simulink model "Energy_Release_System"  (R2022b)
settings: Solver=FixedStepAuto  StartTime=0.0  StopTime=2000  FixedStep=1  RelTol=1e-3
model workspace (MAT data in the model file):
  P0 = 13000
  T0 = 700
  m0 = 30000000
settings Model: Creator=Crapon  LastModifiedBy=Crapon

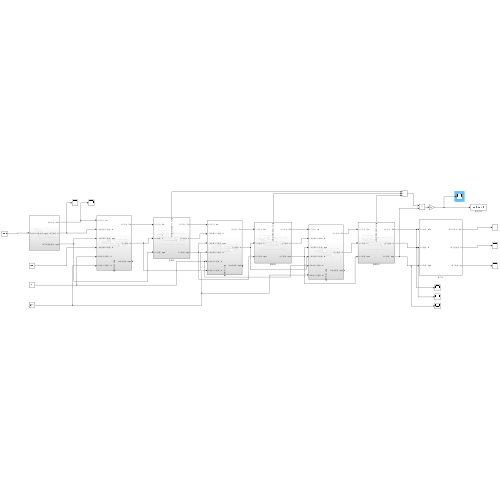
[thumbnail: Simulink's stored preview of the top-level diagram]
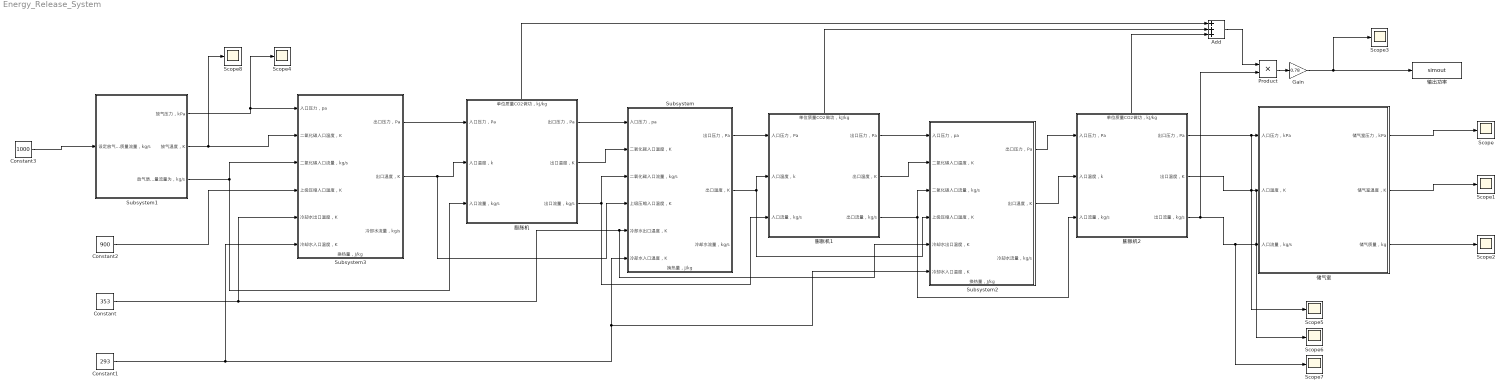
== system Energy_Release_System ==
  Add : Sum  Inputs=+++
  Constant : Constant  Value=353
  Constant1 : Constant  Value=293
  Constant2 : Constant  Value=900
  Constant3 : Constant  Value=1000
  Gain : Gain  Gain=0.78
  Product : Product
  Scope{,1..8} (9 alike) : Scope
  Subsystem : Subsystem
      settings: PortSchema="{\"entries\":[{\"content\":{\"sides\":[{\"content\":{\"connectorIds\":[\"In1\",\"In2\",\"In3\",\"In4\",\"In5\",\"In6\"]},\"type\":\"ConnectorPlacement.EquallySpacedRectSide\",\"uuid\":\"005acfd8-ea89-4894-a254-a05d71797730\"},{\"content\":{\"connectorIds\":[\"Out1\",\"Out2\",\"Out3\"],\"side\":\"RIGHT\"},\"type\":\"ConnectorPlacement.EquallySpacedRectSide\",\"uuid\":\"e66330f7-ec29-462a-8cb5-548756672f09\"},{\"content\":{\"connectorIds\":[],\"side\":\"TOP\"},\"type\":\"ConnectorPlacement.EquallySpacedRectSide\",\"uuid\":\"f5e02eef-e82e-41bc-9a16-8c3a3dd05456\"},{\"content\":{\"connectorIds\":[\"Out4\"],\"side\":\"BOTTOM\"},\"type\":\"ConnectorPlacement.EquallySpacedRectSide\",\"uuid\":\"90480476-9594-4c11-8a2f-3b3d9fc35a98\"}]},\"type\":\"ConnectorPlacement.EquallySpacedConnector\",\"uuid\":\"2499ac2c-0893-45bb-b507-b450c1c8eb76\"}],\"packageUris\":[\"http://schema.mathworks.com/mf0/Connector/R2020b\"],\"version\":\"1.0\"}"
  Subsystem1 : Subsystem
  Subsystem2 : Subsystem
      settings: PortSchema="{\"entries\":[{\"content\":{\"sides\":[{\"content\":{\"connectorIds\":[\"In1\",\"In2\",\"In3\",\"In4\",\"In5\",\"In6\"]},\"type\":\"ConnectorPlacement.EquallySpacedRectSide\",\"uuid\":\"005acfd8-ea89-4894-a254-a05d71797730\"},{\"content\":{\"connectorIds\":[\"Out1\",\"Out2\",\"Out3\"],\"side\":\"RIGHT\"},\"type\":\"ConnectorPlacement.EquallySpacedRectSide\",\"uuid\":\"e66330f7-ec29-462a-8cb5-548756672f09\"},{\"content\":{\"connectorIds\":[],\"side\":\"TOP\"},\"type\":\"ConnectorPlacement.EquallySpacedRectSide\",\"uuid\":\"f5e02eef-e82e-41bc-9a16-8c3a3dd05456\"},{\"content\":{\"connectorIds\":[\"Out4\"],\"side\":\"BOTTOM\"},\"type\":\"ConnectorPlacement.EquallySpacedRectSide\",\"uuid\":\"90480476-9594-4c11-8a2f-3b3d9fc35a98\"}]},\"type\":\"ConnectorPlacement.EquallySpacedConnector\",\"uuid\":\"2499ac2c-0893-45bb-b507-b450c1c8eb76\"}],\"packageUris\":[\"http://schema.mathworks.com/mf0/Connector/R2020b\"],\"version\":\"1.0\"}"
  Subsystem3 : Subsystem
      settings: PortSchema="{\"entries\":[{\"content\":{\"sides\":[{\"content\":{\"connectorIds\":[\"In1\",\"In2\",\"In3\",\"In4\",\"In5\",\"In6\"]},\"type\":\"ConnectorPlacement.EquallySpacedRectSide\",\"uuid\":\"005acfd8-ea89-4894-a254-a05d71797730\"},{\"content\":{\"connectorIds\":[\"Out1\",\"Out2\",\"Out3\"],\"side\":\"RIGHT\"},\"type\":\"ConnectorPlacement.EquallySpacedRectSide\",\"uuid\":\"e66330f7-ec29-462a-8cb5-548756672f09\"},{\"content\":{\"connectorIds\":[],\"side\":\"TOP\"},\"type\":\"ConnectorPlacement.EquallySpacedRectSide\",\"uuid\":\"f5e02eef-e82e-41bc-9a16-8c3a3dd05456\"},{\"content\":{\"connectorIds\":[\"Out4\"],\"side\":\"BOTTOM\"},\"type\":\"ConnectorPlacement.EquallySpacedRectSide\",\"uuid\":\"90480476-9594-4c11-8a2f-3b3d9fc35a98\"}]},\"type\":\"ConnectorPlacement.EquallySpacedConnector\",\"uuid\":\"2499ac2c-0893-45bb-b507-b450c1c8eb76\"}],\"packageUris\":[\"http://schema.mathworks.com/mf0/Connector/R2020b\"],\"version\":\"1.0\"}"
  储气室 : Subsystem
  膨胀机 : Subsystem
      settings: PortSchema="{\"entries\":[{\"content\":{\"sides\":[{\"content\":{\"connectorIds\":[\"In1\",\"In2\",\"In3\"]},\"type\":\"ConnectorPlacement.EquallySpacedRectSide\",\"uuid\":\"af46db4a-1baf-47a9-bc8e-dce7f9faf651\"},{\"content\":{\"connectorIds\":[\"Out1\",\"Out2\",\"Out3\"],\"side\":\"RIGHT\"},\"type\":\"ConnectorPlacement.EquallySpacedRectSide\",\"uuid\":\"0ecd7e62-bca6-4a18-8bf4-9fc15378ff92\"},{\"content\":{\"connectorIds\":[\"Out4\"],\"side\":\"TOP\"},\"type\":\"ConnectorPlacement.EquallySpacedRectSide\",\"uuid\":\"ae3c27ab-cc75-4c7c-b9ef-cea9554166bd\"}]},\"type\":\"ConnectorPlacement.EquallySpacedConnector\",\"uuid\":\"4d6f15aa-483c-4043-8dfd-1170adfd8f34\"}],\"packageUris\":[\"http://schema.mathworks.com/mf0/Connector/R2020b\"],\"version\":\"1.0\"}"
  膨胀机1 : Subsystem
      settings: PortSchema="{\"entries\":[{\"content\":{\"sides\":[{\"content\":{\"connectorIds\":[\"In1\",\"In2\",\"In3\"]},\"type\":\"ConnectorPlacement.EquallySpacedRectSide\",\"uuid\":\"af46db4a-1baf-47a9-bc8e-dce7f9faf651\"},{\"content\":{\"connectorIds\":[\"Out1\",\"Out2\",\"Out3\"],\"side\":\"RIGHT\"},\"type\":\"ConnectorPlacement.EquallySpacedRectSide\",\"uuid\":\"0ecd7e62-bca6-4a18-8bf4-9fc15378ff92\"},{\"content\":{\"connectorIds\":[\"Out4\"],\"side\":\"TOP\"},\"type\":\"ConnectorPlacement.EquallySpacedRectSide\",\"uuid\":\"ae3c27ab-cc75-4c7c-b9ef-cea9554166bd\"}]},\"type\":\"ConnectorPlacement.EquallySpacedConnector\",\"uuid\":\"4d6f15aa-483c-4043-8dfd-1170adfd8f34\"}],\"packageUris\":[\"http://schema.mathworks.com/mf0/Connector/R2020b\"],\"version\":\"1.0\"}"
  膨胀机2 : Subsystem
      settings: PortSchema="{\"entries\":[{\"content\":{\"sides\":[{\"content\":{\"connectorIds\":[\"In1\",\"In2\",\"In3\"]},\"type\":\"ConnectorPlacement.EquallySpacedRectSide\",\"uuid\":\"af46db4a-1baf-47a9-bc8e-dce7f9faf651\"},{\"content\":{\"connectorIds\":[\"Out1\",\"Out2\",\"Out3\"],\"side\":\"RIGHT\"},\"type\":\"ConnectorPlacement.EquallySpacedRectSide\",\"uuid\":\"0ecd7e62-bca6-4a18-8bf4-9fc15378ff92\"},{\"content\":{\"connectorIds\":[\"Out4\"],\"side\":\"TOP\"},\"type\":\"ConnectorPlacement.EquallySpacedRectSide\",\"uuid\":\"ae3c27ab-cc75-4c7c-b9ef-cea9554166bd\"}]},\"type\":\"ConnectorPlacement.EquallySpacedConnector\",\"uuid\":\"4d6f15aa-483c-4043-8dfd-1170adfd8f34\"}],\"packageUris\":[\"http://schema.mathworks.com/mf0/Connector/R2020b\"],\"version\":\"1.0\"}"
  输出功率 : ToWorkspace  VariableName=simout  SaveFormat=Timeseries  SampleTime=-1
  wires:
  Subsystem3/1(出口压力，Pa) -> 膨胀机/1(入口压力，Pa)
  Subsystem3/2(出口温度，K) -> Subsystem/4(上级压缩入口温度，K), 膨胀机/2(入口温度，k)
  Subsystem1/3(放气质量流量为，kg/s) -> Subsystem3/3(二氧化碳入口流量，kg/s), 膨胀机/3(入口流量，kg/s)
  膨胀机/1(出口压力，Pa) -> Subsystem/1(入口压力，pa)
  膨胀机/2(出口温度，K) -> Subsystem/2(二氧化碳入口温度，K)
  膨胀机/3("  出口流量，kg/s") -> Subsystem/3(二氧化碳入口流量，kg/s), 膨胀机1/3(入口流量，kg/s)
  Subsystem/1(出口压力，Pa) -> 膨胀机1/1(入口压力，Pa)
  Subsystem/2(出口温度，K) -> Subsystem2/4(上级压缩入口温度，K), 膨胀机1/2(入口温度，k)
  膨胀机1/1(出口压力，Pa) -> Subsystem2/1(入口压力，pa)
  膨胀机1/2(出口温度，K) -> Subsystem2/2(二氧化碳入口温度，K)
  膨胀机1/3("  出口流量，kg/s") -> 膨胀机2/3(入口流量，kg/s), Subsystem2/3(二氧化碳入口流量，kg/s)
  Subsystem2/1(出口压力，Pa) -> 膨胀机2/1(入口压力，Pa)
  Subsystem2/2(出口温度，K) -> 膨胀机2/2(入口温度，k)
  膨胀机/4(单位质量CO2做功，kJ/kg) -> Add/1
  膨胀机1/4(单位质量CO2做功，kJ/kg) -> Add/2
  膨胀机2/1(出口压力，Pa) -> Scope5/1, 储气室/1(入口压力，kPa)
  膨胀机2/2(出口温度，K) -> Scope6/1, 储气室/2(入口温度，K)
  膨胀机2/3("  出口流量，kg/s") -> Product/2, Scope7/1, 储气室/3(入口流量，kg/s)
  储气室/3(储气质量，kg) -> Scope2/1
  储气室/2(储气室温度，K) -> Scope1/1
  储气室/1(储气室压力，kPa) -> Scope/1
  膨胀机2/4(单位质量CO2做功，kJ/kg) -> Add/3
  Add/1 -> Product/1
  Product/1 -> Gain/1
  Gain/1 -> Scope3/1, 输出功率/1
  Constant/1 -> Subsystem3/5(冷却水出口温度，K), Subsystem2/5(冷却水出口温度，K), Subsystem/5(冷却水出口温度，K)
  Constant1/1 -> Subsystem3/6(冷却水入口温度，K), Subsystem2/6(冷却水入口温度，K), Subsystem/6(冷却水入口温度，K)
  Constant2/1 -> Subsystem3/4(上级压缩入口温度，K)
  Subsystem1/1(放气压力，kPa) -> Scope4/1, Subsystem3/1(入口压力，pa)
  Subsystem1/2(放气温度，K) -> Scope8/1, Subsystem3/2(二氧化碳入口温度，K)
  Constant3/1 -> Subsystem1/1(设定放气质量流量，kg/s)

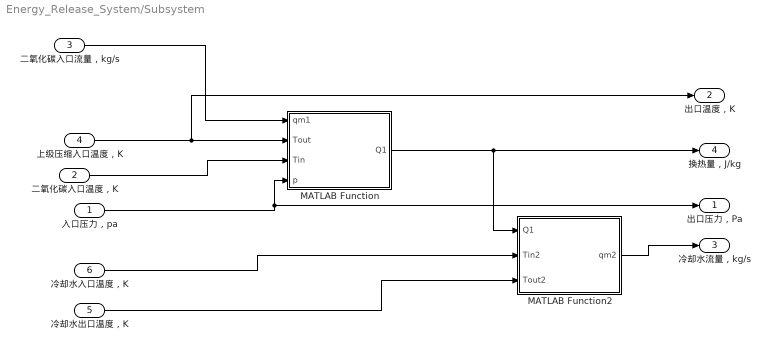
== system Energy_Release_System/Subsystem ==
  入口压力，pa : Inport
  二氧化碳入口温度，K : Inport  Port=2
  二氧化碳入口流量，kg/s : Inport  Port=3
  上级压缩入口温度，K : Inport  Port=4
  冷却水出口温度，K : Inport  Port=5
  冷却水入口温度，K : Inport  Port=6
  MATLAB Function : MATLAB Function  TreatAsAtomicUnit=on
  MATLAB Function2 : MATLAB Function  TreatAsAtomicUnit=on
  出口压力，Pa : Outport
  出口温度，K : Outport  Port=2
  冷却水流量，kg/s : Outport  Port=3
  换热量，J/kg : Outport  Port=4
  wires:
  MATLAB Function/1(Q1) -> 换热量，J/kg/1, MATLAB Function2/1(Q1)
  冷却水出口温度，K/1 -> MATLAB Function2/3(Tout2)
  冷却水入口温度，K/1 -> MATLAB Function2/2(Tin2)
  MATLAB Function2/1(qm2) -> 冷却水流量，kg/s/1
  二氧化碳入口温度，K/1 -> MATLAB Function/3(Tin)
  上级压缩入口温度，K/1 -> 出口温度，K/1, MATLAB Function/2(Tout)
  二氧化碳入口流量，kg/s/1 -> MATLAB Function/1(qm1)
  入口压力，pa/1 -> MATLAB Function/4(p), 出口压力，Pa/1

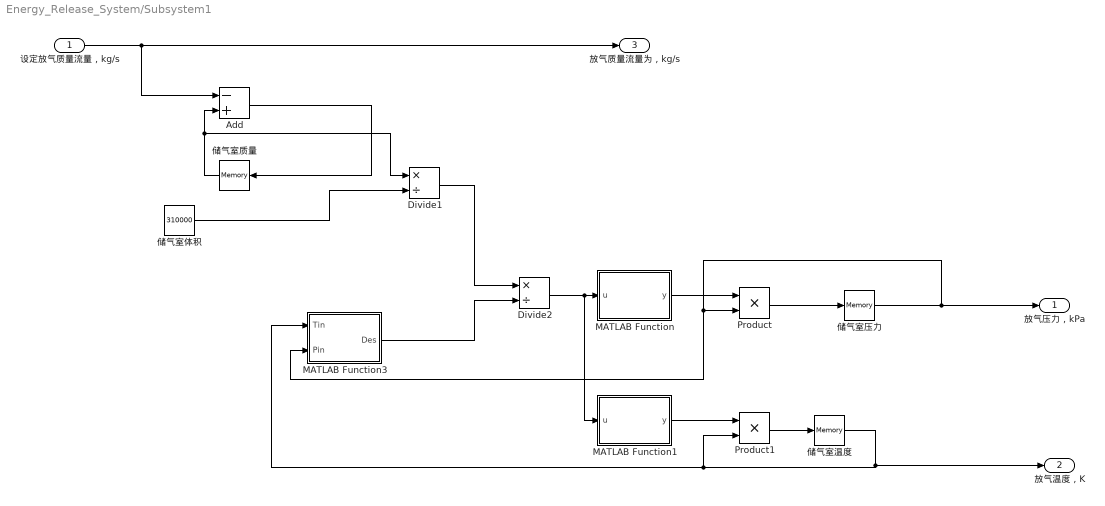
== system Energy_Release_System/Subsystem1 ==
  设定放气质量流量，kg/s : Inport
  Add : Sum  Inputs=-+
  Divide1 : Product  Inputs=*/
  Divide2 : Product  Inputs=*/
  MATLAB Function : MATLAB Function  TreatAsAtomicUnit=on
  MATLAB Function1 : MATLAB Function  TreatAsAtomicUnit=on
  MATLAB Function3 : MATLAB Function  TreatAsAtomicUnit=on
  Product : Product
  Product1 : Product
  储气室体积 : Constant  Value=310000
  储气室压力 : Memory  InitialCondition=P0
  储气室温度 : Memory  InitialCondition=T0
  储气室质量 : Memory  InitialCondition=m0
  放气压力，kPa : Outport
  放气温度，K : Outport  Port=2
  放气质量流量为，kg/s : Outport  Port=3
  wires:
  设定放气质量流量，kg/s/1 -> 放气质量流量为，kg/s/1, Add/1
  MATLAB Function3/1(Des) -> Divide2/2
  储气室质量/1 -> Divide1/1, Add/2
  Add/1 -> 储气室质量/1
  储气室体积/1 -> Divide1/2
  Divide1/1 -> Divide2/1
  Divide2/1 -> MATLAB Function1/1(u), MATLAB Function/1(u)
  储气室压力/1 -> Product/2, MATLAB Function3/2(Pin), 放气压力，kPa/1
  Product/1 -> 储气室压力/1
  MATLAB Function1/1(y) -> Product1/1
  Product1/1 -> 储气室温度/1
  储气室温度/1 -> MATLAB Function3/1(Tin), Product1/2, 放气温度，K/1
  MATLAB Function/1(y) -> Product/1

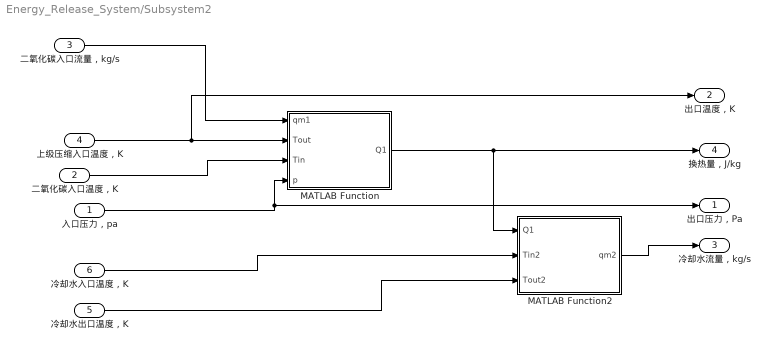
== system Energy_Release_System/Subsystem2 ==
  入口压力，pa : Inport
  二氧化碳入口温度，K : Inport  Port=2
  二氧化碳入口流量，kg/s : Inport  Port=3
  上级压缩入口温度，K : Inport  Port=4
  冷却水出口温度，K : Inport  Port=5
  冷却水入口温度，K : Inport  Port=6
  MATLAB Function : MATLAB Function  TreatAsAtomicUnit=on
  MATLAB Function2 : MATLAB Function  TreatAsAtomicUnit=on
  出口压力，Pa : Outport
  出口温度，K : Outport  Port=2
  冷却水流量，kg/s : Outport  Port=3
  换热量，J/kg : Outport  Port=4
  wires:
  入口压力，pa/1 -> 出口压力，Pa/1, MATLAB Function/4(p)
  二氧化碳入口流量，kg/s/1 -> MATLAB Function/1(qm1)
  上级压缩入口温度，K/1 -> MATLAB Function/2(Tout), 出口温度，K/1
  二氧化碳入口温度，K/1 -> MATLAB Function/3(Tin)
  MATLAB Function2/1(qm2) -> 冷却水流量，kg/s/1
  冷却水入口温度，K/1 -> MATLAB Function2/2(Tin2)
  冷却水出口温度，K/1 -> MATLAB Function2/3(Tout2)
  MATLAB Function/1(Q1) -> MATLAB Function2/1(Q1), 换热量，J/kg/1

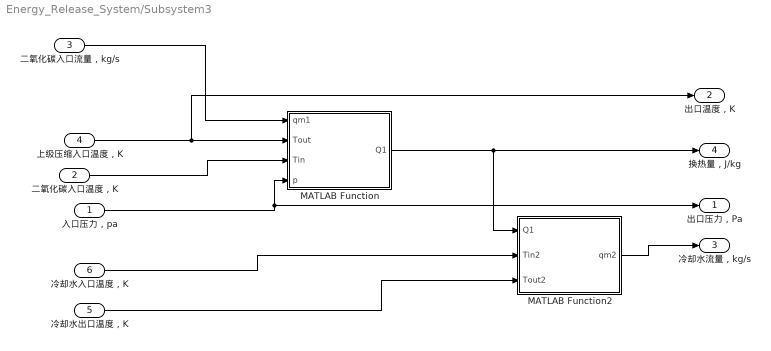
== system Energy_Release_System/Subsystem3 ==
  入口压力，pa : Inport
  二氧化碳入口温度，K : Inport  Port=2
  二氧化碳入口流量，kg/s : Inport  Port=3
  上级压缩入口温度，K : Inport  Port=4
  冷却水出口温度，K : Inport  Port=5
  冷却水入口温度，K : Inport  Port=6
  MATLAB Function : MATLAB Function  TreatAsAtomicUnit=on
  MATLAB Function2 : MATLAB Function  TreatAsAtomicUnit=on
  出口压力，Pa : Outport
  出口温度，K : Outport  Port=2
  冷却水流量，kg/s : Outport  Port=3
  换热量，J/kg : Outport  Port=4
  wires:
  入口压力，pa/1 -> 出口压力，Pa/1, MATLAB Function/4(p)
  二氧化碳入口流量，kg/s/1 -> MATLAB Function/1(qm1)
  上级压缩入口温度，K/1 -> MATLAB Function/2(Tout), 出口温度，K/1
  二氧化碳入口温度，K/1 -> MATLAB Function/3(Tin)
  MATLAB Function2/1(qm2) -> 冷却水流量，kg/s/1
  冷却水入口温度，K/1 -> MATLAB Function2/2(Tin2)
  冷却水出口温度，K/1 -> MATLAB Function2/3(Tout2)
  MATLAB Function/1(Q1) -> MATLAB Function2/1(Q1), 换热量，J/kg/1

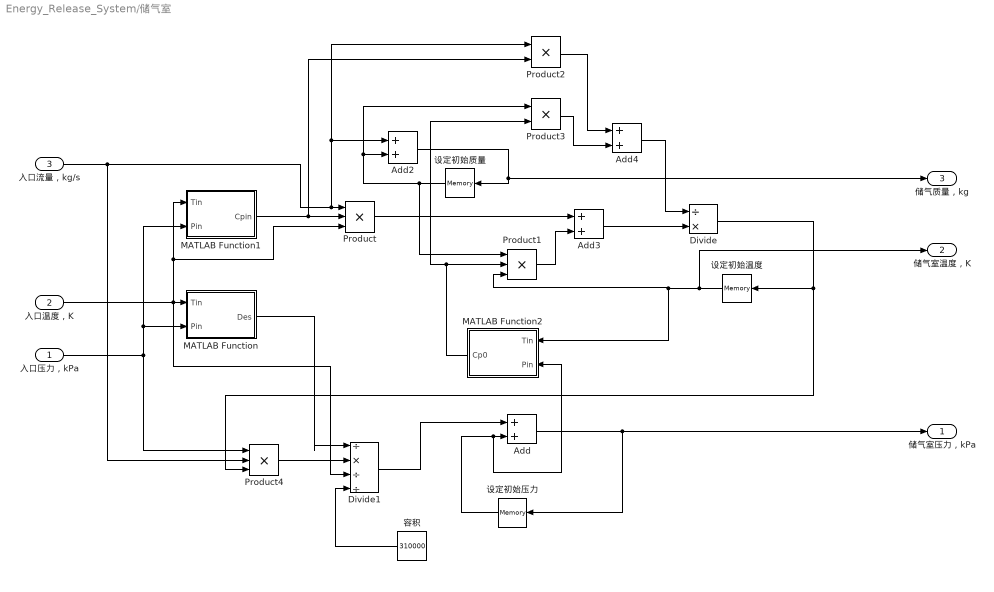
== system Energy_Release_System/储气室 ==
  入口压力，kPa : Inport
  入口温度，K : Inport  Port=2
  入口流量，kg/s : Inport  Port=3
  Add{,2..4} (4 alike) : Sum
  Divide : Product  Inputs=/*
  Divide1 : Product  Inputs=/*//
  MATLAB Function : MATLAB Function  TreatAsAtomicUnit=on
  MATLAB Function1 : MATLAB Function  TreatAsAtomicUnit=on
  MATLAB Function2 : MATLAB Function  TreatAsAtomicUnit=on
  Product : Product  Inputs=3
  Product1 : Product  Inputs=3
  Product2 : Product
  Product3 : Product
  Product4 : Product  Inputs=3
  容积 : Constant  Value=310000
  设定初始压力 : Memory  InitialCondition=100
  设定初始温度 : Memory  InitialCondition=300
  设定初始质量 : Memory  InitialCondition=320000
  储气室压力，kPa : Outport
  储气室温度，K : Outport  Port=2
  储气质量，kg : Outport  Port=3
  wires:
  入口流量，kg/s/1 -> Product4/2, Product2/1, Add2/1, Product/1
  设定初始质量/1 -> Product1/1, Product3/1, Add2/2
  Product2/1 -> Add4/1
  MATLAB Function1/1(Cpin) -> Product/2, Product2/2
  Product4/1 -> Divide1/2
  MATLAB Function2/1(Cp0) -> Product1/2, Product3/2
  Divide1/1 -> Add/1
  入口温度，K/1 -> MATLAB Function1/1(Tin), Product/3, MATLAB Function/1(Tin), Divide1/3
  Product1/1 -> Add3/2
  Add/1 -> 储气室压力，kPa/1, 设定初始压力/1
  入口压力，kPa/1 -> Product4/1, MATLAB Function1/2(Pin), MATLAB Function/2(Pin)
  Add4/1 -> Divide/1
  设定初始压力/1 -> MATLAB Function2/2(Pin), Add/2
  容积/1 -> Divide1/4
  Product3/1 -> Add4/2
  MATLAB Function/1(Des) -> Divide1/1
  Add3/1 -> Divide/2
  Product/1 -> Add3/1
  Divide/1 -> Product4/3, 设定初始温度/1
  Add2/1 -> 设定初始质量/1, 储气质量，kg/1
  设定初始温度/1 -> 储气室温度，K/1, MATLAB Function2/1(Tin), Product1/3

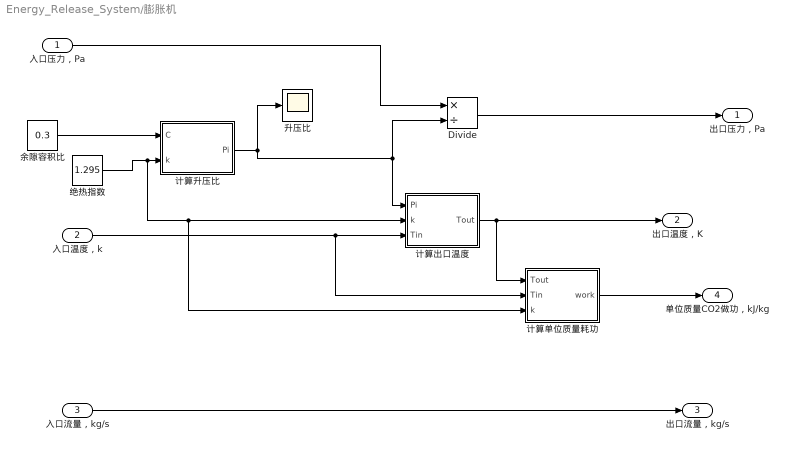
== system Energy_Release_System/膨胀机 ==
  入口压力，Pa : Inport
  入口温度，k : Inport  Port=2
  入口流量，kg/s : Inport  Port=3
  Divide : Product  Inputs=*/
  余隙容积比 : Constant  Value=0.3
  升压比 : Scope
  绝热指数 : Constant  Value=1.295
  计算出口温度 : MATLAB Function  TreatAsAtomicUnit=on
  计算升压比 : MATLAB Function  TreatAsAtomicUnit=on
  计算单位质量耗功 : MATLAB Function  TreatAsAtomicUnit=on
  出口压力，Pa : Outport
  出口温度，K : Outport  Port=2
  "  出口流量，kg/s" : Outport  Port=3
  单位质量CO2做功，kJ/kg : Outport  Port=4
  wires:
  余隙容积比/1 -> 计算升压比/1(C)
  入口压力，Pa/1 -> Divide/1
  绝热指数/1 -> 计算单位质量耗功/3(k), 计算出口温度/2(k), 计算升压比/2(k)
  Divide/1 -> 出口压力，Pa/1
  计算单位质量耗功/1(work) -> 单位质量CO2做功，kJ/kg/1
  计算升压比/1(Pi) -> Divide/2, 计算出口温度/1(Pi), 升压比/1
  入口温度，k/1 -> 计算单位质量耗功/2(Tin), 计算出口温度/3(Tin)
  计算出口温度/1(Tout) -> 出口温度，K/1, 计算单位质量耗功/1(Tout)
  入口流量，kg/s/1 -> "  出口流量，kg/s"/1

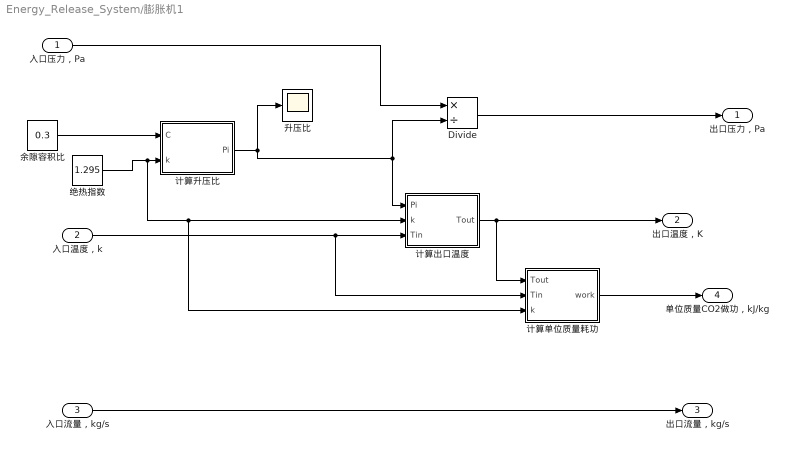
== system Energy_Release_System/膨胀机1 ==
  入口压力，Pa : Inport
  入口温度，k : Inport  Port=2
  入口流量，kg/s : Inport  Port=3
  Divide : Product  Inputs=*/
  余隙容积比 : Constant  Value=0.3
  升压比 : Scope
  绝热指数 : Constant  Value=1.295
  计算出口温度 : MATLAB Function  TreatAsAtomicUnit=on
  计算升压比 : MATLAB Function  TreatAsAtomicUnit=on
  计算单位质量耗功 : MATLAB Function  TreatAsAtomicUnit=on
  出口压力，Pa : Outport
  出口温度，K : Outport  Port=2
  "  出口流量，kg/s" : Outport  Port=3
  单位质量CO2做功，kJ/kg : Outport  Port=4
  wires:
  入口流量，kg/s/1 -> "  出口流量，kg/s"/1
  计算出口温度/1(Tout) -> 计算单位质量耗功/1(Tout), 出口温度，K/1
  入口温度，k/1 -> 计算出口温度/3(Tin), 计算单位质量耗功/2(Tin)
  计算升压比/1(Pi) -> 升压比/1, 计算出口温度/1(Pi), Divide/2
  计算单位质量耗功/1(work) -> 单位质量CO2做功，kJ/kg/1
  Divide/1 -> 出口压力，Pa/1
  绝热指数/1 -> 计算升压比/2(k), 计算出口温度/2(k), 计算单位质量耗功/3(k)
  入口压力，Pa/1 -> Divide/1
  余隙容积比/1 -> 计算升压比/1(C)

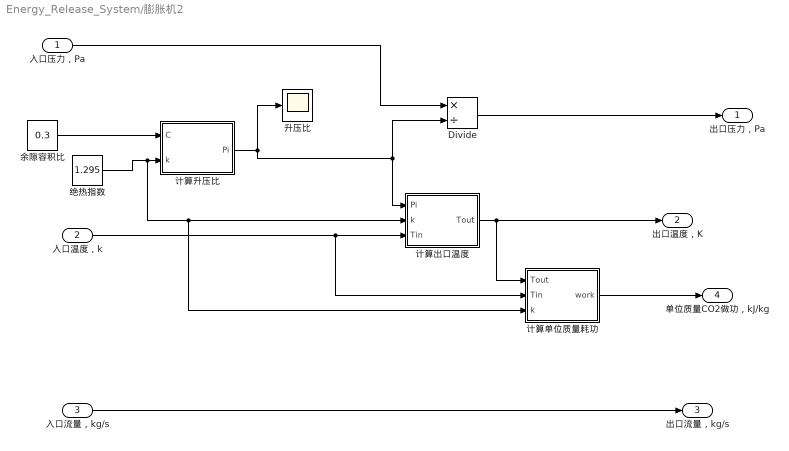
== system Energy_Release_System/膨胀机2 ==
  入口压力，Pa : Inport
  入口温度，k : Inport  Port=2
  入口流量，kg/s : Inport  Port=3
  Divide : Product  Inputs=*/
  余隙容积比 : Constant  Value=0.3
  升压比 : Scope
  绝热指数 : Constant  Value=1.295
  计算出口温度 : MATLAB Function  TreatAsAtomicUnit=on
  计算升压比 : MATLAB Function  TreatAsAtomicUnit=on
  计算单位质量耗功 : MATLAB Function  TreatAsAtomicUnit=on
  出口压力，Pa : Outport
  出口温度，K : Outport  Port=2
  "  出口流量，kg/s" : Outport  Port=3
  单位质量CO2做功，kJ/kg : Outport  Port=4
  wires:
  余隙容积比/1 -> 计算升压比/1(C)
  入口压力，Pa/1 -> Divide/1
  绝热指数/1 -> 计算单位质量耗功/3(k), 计算出口温度/2(k), 计算升压比/2(k)
  Divide/1 -> 出口压力，Pa/1
  计算单位质量耗功/1(work) -> 单位质量CO2做功，kJ/kg/1
  计算升压比/1(Pi) -> Divide/2, 计算出口温度/1(Pi), 升压比/1
  入口温度，k/1 -> 计算单位质量耗功/2(Tin), 计算出口温度/3(Tin)
  计算出口温度/1(Tout) -> 出口温度，K/1, 计算单位质量耗功/1(Tout)
  入口流量，kg/s/1 -> "  出口流量，kg/s"/1

== matlab function Energy_Release_System/Subsystem1/MATLAB Function3 ==
  data: Tin input; Des output; Pin input
function Des = fcn(Tin,Pin)
coder.extrinsic('refpropm');
Des=zeros(1);
Des = refpropm('D','T',Tin,'P',Pin,'CO2');

== matlab function Energy_Release_System/膨胀机/计算出口温度 ==
  data: Pi input; Tout output; k input; Tin input
function Tout= fcn(Pi, k, Tin)

Tout=Tin/((Pi)^((k-1)/k));

== matlab function Energy_Release_System/Subsystem/MATLAB Function ==
  data: qm1 input; Tout input; Tin input; Q1 output; p input
function Q1 = fc(qm1,Tout,Tin,p)
coder.extrinsic('refpropm');
cp=zeros(1);
t=(Tin+Tout)/2;
cp=refpropm('C','T',t,'P',p,'CO2');
Q1= qm1*cp*(Tout-Tin);

== matlab function Energy_Release_System/Subsystem/MATLAB Function2 ==
  data: Q1 input; Tin2 input; Tout2 input; qm2 output
function qm2 = fcn(Q1,Tin2,Tout2)
coder.extrinsic('refpropm');
cp=zeros(1);
t=(Tin2+Tout2)/2;
cp=refpropm('C','T',t,'Q',0,'water');
qm2= Q1/(cp*(Tout2-Tin2));

== matlab function Energy_Release_System/膨胀机2/计算升压比 ==
  data: C input; Pi output; k input
function Pi = fcn(C, k)

Pi =(1+1/C)^k;

== matlab function Energy_Release_System/膨胀机2/计算单位质量耗功 ==
  data: Tout input; Tin input; k input; work output
function work= fcn(Tout,Tin,k)
Rg=0.189;
work=(k/(k-1))*Rg*(-Tout+Tin);

== matlab function Energy_Release_System/储气室/MATLAB Function ==
  data: Tin input; Des output; Pin input
function Des = fcn(Tin,Pin)
coder.extrinsic('refpropm');
Des=zeros(1);
Des = refpropm('D','T',Tin,'P',Pin,'CO2');

== matlab function Energy_Release_System/储气室/MATLAB Function1 ==
  data: Tin input; Cpin output; Pin input
function Cpin = fcn(Tin,Pin)
coder.extrinsic('refpropm');
Cpin=zeros(1);
Cpin = refpropm('C','T',Tin,'P',Pin,'CO2');

== matlab function Energy_Release_System/储气室/MATLAB Function2 ==
  data: Tin input; Cp0 output; Pin input
function Cp0 = fcn(Tin,Pin)
coder.extrinsic('refpropm');
Cp0=zeros(1);
Cp0 = refpropm('C','T',Tin,'P',Pin,'CO2');

== matlab function Energy_Release_System/Subsystem3/MATLAB Function ==
  data: qm1 input; Tout input; Tin input; Q1 output; p input
function Q1 = fc(qm1,Tout,Tin,p)
t=(Tin+Tout)/2;
coder.extrinsic('refpropm');
cp=zeros(1);
cp=refpropm('C','T',t,'P',p,'CO2');
Q1= qm1*cp*(Tout-Tin);

== matlab function Energy_Release_System/Subsystem3/MATLAB Function2 ==
  data: Q1 input; Tin2 input; Tout2 input; qm2 output
function qm2 = fcn(Q1,Tin2,Tout2)
t=(Tin2+Tout2)/2;
coder.extrinsic('refpropm');
cp=zeros(1);
cp=refpropm('C','T',t,'Q',0,'water');
qm2= Q1/(cp*(Tout2-Tin2));

== matlab function Energy_Release_System/膨胀机/计算单位质量耗功 ==
  data: Tout input; Tin input; k input; work output
function work= fcn(Tout,Tin,k)
Rg=0.189;
work=(k/(k-1))*Rg*(-Tout+Tin);

== matlab function Energy_Release_System/膨胀机1/计算出口温度 ==
  data: Pi input; Tout output; k input; Tin input
function Tout= fcn(Pi, k, Tin)

Tout=Tin/((Pi)^((k-1)/k));

== matlab function Energy_Release_System/膨胀机/计算升压比 ==
  data: C input; Pi output; k input
function Pi = fcn(C, k)

Pi =(1+1/C)^k;

== matlab function Energy_Release_System/膨胀机1/计算升压比 ==
  data: C input; Pi output; k input
function Pi = fcn(C, k)

Pi =(1+1/C)^k;

== matlab function Energy_Release_System/膨胀机1/计算单位质量耗功 ==
  data: Tout input; Tin input; k input; work output
function work= fcn(Tout,Tin,k)
Rg=0.189;
work=(k/(k-1))*Rg*(-Tout+Tin);

== matlab function Energy_Release_System/Subsystem2/MATLAB Function ==
  data: qm1 input; Tout input; Tin input; Q1 output; p input
function Q1 = fc(qm1,Tout,Tin,p)
t=(Tin+Tout)/2;
coder.extrinsic('refpropm');
cp=zeros(1);
cp=refpropm('C','T',t,'P',p,'CO2');
Q1= qm1*cp*(Tout-Tin);

== matlab function Energy_Release_System/Subsystem2/MATLAB Function2 ==
  data: Q1 input; Tin2 input; Tout2 input; qm2 output
function qm2 = fcn(Q1,Tin2,Tout2)
t=(Tin2+Tout2)/2;
coder.extrinsic('refpropm');
cp=zeros(1);
cp=refpropm('C','T',t,'Q',0,'water');
qm2= Q1/(cp*(Tout2-Tin2));

== matlab function Energy_Release_System/膨胀机2/计算出口温度 ==
  data: Pi input; Tout output; k input; Tin input
function Tout= fcn(Pi, k, Tin)

Tout=Tin/((Pi)^((k-1)/k));

== matlab function Energy_Release_System/Subsystem1/MATLAB Function ==
  data: u input; y output
function y = fcn(u)

y = u^1.295;

== matlab function Energy_Release_System/Subsystem1/MATLAB Function1 ==
  data: u input; y output
function y = fcn(u)

y = u^0.295;
